simulink model "PanelSolarSeguidor_mk2_comp"  (R2022a)
settings: Solver=VariableStepAuto  StartTime=0.0  StopTime=14  RelTol=1e-3
model workspace (MAT data in the model file):
  Sig = Simulink.Signal
  Sig.DataType = 'auto'
  Sig.DocUnits = 'deg'
  Sig.Dimensions = -1
  Sig.DimensionsMode = 'auto'
  Sig.Complexity = 'auto'
  Sig.SampleTime = -1
  Sig.SamplingMode = 'auto'
values from neighbouring files (symbols this model uses):
  dia = 1    [PanelSolarSeguidor_3D.m]
  dph = 0.35    [PanelSolarSeguidor_3D.m]
  eficiencia_custom = 10    [PanelSolarSeguidor_3D.m]
  G_retroceso = -20    [PanelSolarSeguidor_3D.m]
  hra = 1    [PanelSolarSeguidor_3D.m]
  Kd = 5    [PanelSolarSeguidor.mat]    (also in PanelSolarSeguidor_3D.m)
  Kf = 1.835    [PanelSolarSeguidor.mat]    (also in PanelSolarSeguidor_3D.m)
  Kg = 20    [PanelSolarSeguidor.mat]    (also in PanelSolarSeguidor_3D.m)
  Kt = 1.835    [PanelSolarSeguidor.mat]    (also in PanelSolarSeguidor_3D.m)
  L = 0.1042    [PanelSolarSeguidor.mat]    (also in PanelSolarSeguidor_3D.m)
  latitud = -36.83078129680368    (= -36.8307812968)    [PanelSolarSeguidor_3D.m]
  longitud = -73.0368870295651    (= -73.0368870296)    [PanelSolarSeguidor_3D.m]
  m = 24.5    [PanelSolarSeguidor.mat]
  mes = 1    [PanelSolarSeguidor_3D.m]
  mn = 0    [PanelSolarSeguidor_3D.m]
  P_L = 2.18    [PanelSolarSeguidor_3D.m]
  P_W = 0.996    [PanelSolarSeguidor_3D.m]
  R = 3.05    [PanelSolarSeguidor.mat]    (also in PanelSolarSeguidor_3D.m)
  S_l = 0.2    [PanelSolarSeguidor_3D.m]
  S_w = 0.1    [PanelSolarSeguidor_3D.m]
  secs = 0    [PanelSolarSeguidor_3D.m]
  selector_eficiencia = 0    [PanelSolarSeguidor_3D.m]
  timezone = -3    [PanelSolarSeguidor_3D.m]
libraries: simulink x21, simulink_extras x9, slpidlib x2
settings Model: Creator=marte  LastModifiedBy=fmartel2019
settings ModelReferenceCC: EnableRefExpFcnMdlSchedulingChecks=off
settings RTWCC: Description=Generic Real-Time Target

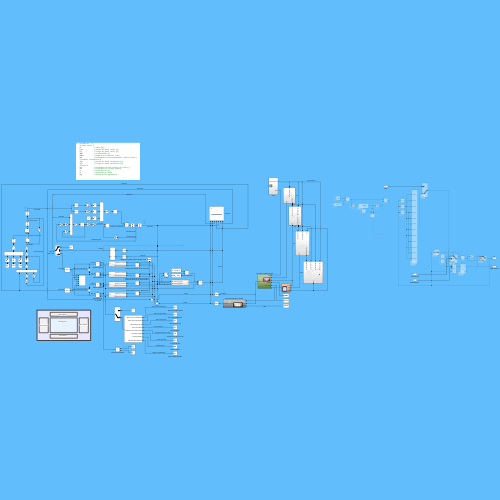
[thumbnail: Simulink's stored preview of the top-level diagram]
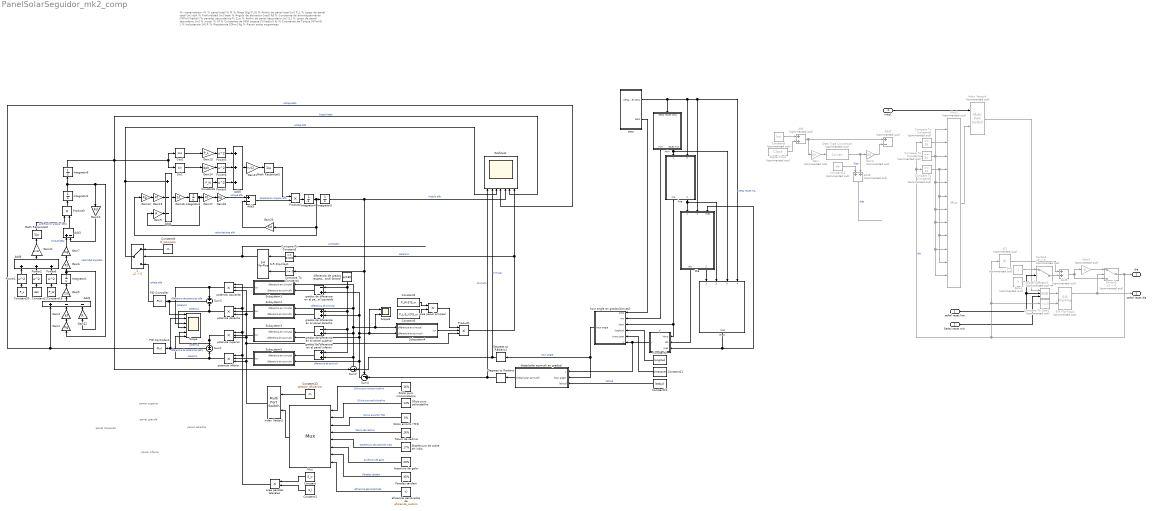
== system PanelSolarSeguidor_mk2_comp ==
  note: %---parametros---%
      | % panel total %
      | M % Masa [Kg]
      | P_W % Ancho de panel total [m]
      | P_L % Largo de panel total [m]
      | dph % Profundidad [m]
      | beta % Ángulo de elevación [rad]
      | Kd % Constante de amortiguamiento [(N*m)/(rad/s)]
      | %-paneles secundarios-%
      | S_w % Ancho de panel secundario [m]
      | S_l % Largo de panel secundario [m]
      | % motor %
      | Kf % Constante de FEM trasera [V/(rad/s)]
      | Kt % Constante de Torque [N*m/A]
      | L % Inductancia [H]
      | R % Resistencia [Ohm]
      | Kg % Razón entre engranajes
  note: panel superior
  note: panel inferior
  note: panel derecho
  note: panel izquierdo
  note: panel grande
  señal reset hra : Inport
  Señal reset min : Inport  Port=2
  mes1 : Inport  Port=3
  1 : Switch  Criteria=u2 > Threshold  SaturateOnIntegerOverflow=off  InputSameDT=off
  Add : Sum  Commented=on
  Add1 : Sum  Inputs=+-
  Add2 : Sum  Inputs=+--
  Add3 : Sum  Inputs=+-
  Add4 : Sum  Inputs=+--
  Add5 : Sum  Inputs=+++
  Add6 : Sum  Inputs=+++
  Add7 : Sum  Commented=on  Inputs=+-
  Add8 : Sum  Commented=on
  Add9 : Sum  Commented=on
  "Arseniuro de galio " : Constant  Value=20%
  Compare To Constant3 : simulink/Logic and Bit Operations/Compare To Constant  Commented=on  relop===  const=31  OutDataTypeStr=boolean
  Compare To Constant4 : simulink/Logic and Bit Operations/Compare To Constant  relop=<=  const=0  OutDataTypeStr=boolean
  Compare To Constant5 : simulink/Logic and Bit Operations/Compare To Constant  relop=<=  const=0.001  OutDataTypeStr=boolean
  Compare To Constant6 : simulink/Logic and Bit Operations/Compare To Constant  Commented=on  relop===  const=28  OutDataTypeStr=boolean
  Compare To Constant8 : simulink/Logic and Bit Operations/Compare To Constant  Commented=on  relop===  const=31  OutDataTypeStr=boolean
  Compare To Zero2 : simulink/Logic and Bit Operations/Compare To Zero  Commented=on  relop=<=  OutDataTypeStr=boolean
  Constant : Constant  Value=S_w
  Constant1 : Constant  Value=S_l
  Constant10 : Constant  Value=latitud
  Constant11 : Constant  Value=timezone
  Constant12 : Constant  Commented=on  Value=dia
  Constant13 : Constant  Value=selector_eficiencia
  Constant19 : Constant  Value=P_W
  Constant2 : Constant  Value=P_W-2*S_w
  Constant20 : Constant  Value=P_L
  Constant23 : Constant  Value=dph
  Constant3 : Constant  Value=P_L-S_l-2*S_w
  Constant4 : Constant  Value=longitud
  Constant5 : Constant  Commented=on  Value=hra
  Constant6 : Constant  Value=P_W
  Constant9 : Constant  Value=G_retroceso
  Cos1 : Trigonometry  Operator=cos
  Data Type Conversion : DataTypeConversion  Commented=on  SaturateOnIntegerOverflow=off  RndMeth=Floor
  Degrees to Radians : simulink_extras/Transformations/Degrees to Radians
  Degrees to Radians1 : simulink_extras/Transformations/Degrees to Radians
  Dia : Subsystem
  Digital Clock : DigitalClock  Commented=on
  Diseleniuro de cobre en indio : Constant  Value=17%
  Gain : Gain  Commented=on  Gain=1/24
  Gain{1,7,12,18} (4 alike) : Gain  Gain=Kg
  Gain10 : Gain  Gain=Kd
  Gain11 : Gain  Gain=m/12
  Gain13 : Gain  Gain=P_L
  Gain14 : Gain  Gain=dph
  Gain15 : Gain  Gain=Kf
  Gain16 : Gain  Gain=1/L
  Gain17 : Gain  Gain=Kt
  Gain2 : Gain  Commented=on  Gain=24
  Gain20 : Gain  Gain=Kd
  Gain21 : Gain  Gain=m/12
  Gain22 : Gain  Gain=R
  Gain3 : Gain  Commented=on  Gain=0
  Gain4 : Gain  Gain=Kf
  Gain5 : Gain  Gain=1/L
  Gain6 : Gain  Gain=Kt
  Gain9 : Gain  Gain=R
  Graficos1 : Scope  NumInputPorts=7
  IC2 : InitialCondition  Commented=on  Value=dia
  Index Vector2 : MultiPortSwitch  DataPortOrder=Zero-based contiguous  Inputs=1  zeroidx=on  SaturateOnIntegerOverflow=off  InputSameDT=off
  Index Vector4 : MultiPortSwitch  Commented=on  DataPortOrder=Zero-based contiguous  Inputs=1  zeroidx=on  SaturateOnIntegerOverflow=off  InputSameDT=off
  Integrator{1..6} (6 alike) : Integrator
  Logical Operator1 : Logic  Commented=on  Inputs=3  AllPortsSameDT=off  OutDataTypeStr=boolean
  Math Reciprocal1 : Math  Operator=reciprocal  SignedPower=on
  Math Reciprocal2 : Math  Operator=reciprocal  SignedPower=on
  Mux : Mux  Inputs=8
      settings: DisplayOption=signals
  Mux3 : Mux  Commented=on  Inputs=12
      settings: DisplayOption=signals
  One : Constant  Commented=on  OutDataTypeStr=Inherit: Inherit via back propagation
  PID Controller : slpidlib/PID Controller  Controller=P  Form=Parallel  TimeDomain=Continuous-time  UseExternalTs=off  SampleTime=-1  IntegratorMethod=Forward Euler  FilterMethod=Forward Euler  ControllerParametersSource=internal  P=10  I=0  UseKiTs=off  D=15  N=100  UseFilter=on  TunerSelectOption=Transfer Function Based (PID Tuner App)  InitialConditionSource=internal  InitialConditionForIntegrator=0  InitialConditionForFilter=0  DifferentiatorICPrevScaledInput=0  ExternalReset=none  TrackingMode=off  Kt=1  LimitOutput=off  SatLimitsSource=internal  UpperSaturationLimit=inf  LowerSaturationLimit=-inf  LinearizeAsGain=on  AntiWindupMode=none  Kb=1  POutMin=[]  POutMax=[]  IOutMin=[]  IOutMax=[]  DOutMin=[]  DOutMax=[]  NOutMin=[]  NOutMax=[]  SumOutMin=[]  SumOutMax=[]  SaturationOutMin=[]  SaturationOutMax=[]  PParamMin=[]  PParamMax=[]  IParamMin=[]  IParamMax=[]  DParamMin=[]  DParamMax=[]  NParamMin=[]  NParamMax=[]  KbParamMin=[]  KbParamMax=[]  KtParamMin=[]  KtParamMax=[]  KbOutMin=[]  KbOutMax=[]  KtOutMin=[]  KtOutMax=[]  IntegratorOutMin=[]  IntegratorOutMax=[]  FilterOutMin=[]  FilterOutMax=[]  SumI1OutMin=[]  SumI1OutMax=[]  SumI2OutMin=[]  SumI2OutMax=[]  SumI3OutMin=[]  SumI3OutMax=[]  SumI4OutMin=[]  SumI4OutMax=[]  SumDOutMin=[]  SumDOutMax=[]  DifferentiatorOutMin=[]  DifferentiatorOutMax=[]  FilterDiffOutCoefMin=[]  FilterDiffOutCoefMax=[]  ReciprocalOutMin=[]  ReciprocalOutMax=[]  SumDenOutMin=[]  SumDenOutMax=[]  SumNumOutMin=[]  SumNumOutMax=[]  DivideOutMin=[]  DivideOutMax=[]  UdiffTsProdOutMin=[]  UdiffTsProdOutMax=[]  NTsProdOutMin=[]  NTsProdOutMax=[]  UintegralTsProdOutMin=[]  UintegralTsProdOutMax=[]  UngainTsProdOutMin=[]  UngainTsProdOutMax=[]  IntegratorContinuousStateAttributes=''  IntegratorStateMustResolveToSignalObject=off  IntegratorRTWStateStorageClass=Auto  FilterContinuousStateAttributes=''  FilterStateMustResolveToSignalObject=off  FilterRTWStateStorageClass=Auto  ParallelPVariant=InternalParameters  IdealPVariant=Disabled  IVariant=Disabled  DVariant=Disabled  IntegratorVariant=Disabled  SatVariant=Disabled  AWVariant=Disabled  PCopyVariant=Disabled  TRVariant=Disabled  FdbkBlocksVariant=Forward  IdealPFdbkVariant=Disabled  SatFdbkVariant=Disabled  DerivativeFilterVariant=Disabled  NVariant=Disabled  NCopyVariant=Disabled_SignalSpec  FilterICVariant=Disabled  IntegratorICVariant=Disabled  ExternalResetVariant=Disabled  TRSumVariant=Passthrough  SumFdbkVariant=Disabled  SumVariant=Passthrough_P  TsampFilterVariant=InternalTs  TsampNgainVariant=Passthrough  TsampIntegralVariant=Disabled_SignalSpec  ExternalSaturationOutDataTypeStr=Inherit: Same as second input  aMode=0
  PID Controller1 : slpidlib/PID Controller  Controller=P  Form=Parallel  TimeDomain=Continuous-time  UseExternalTs=off  SampleTime=-1  IntegratorMethod=Forward Euler  FilterMethod=Forward Euler  ControllerParametersSource=internal  P=1  I=0  UseKiTs=off  D=0  N=100  UseFilter=on  TunerSelectOption=Transfer Function Based (PID Tuner App)  InitialConditionSource=internal  InitialConditionForIntegrator=0  InitialConditionForFilter=0  DifferentiatorICPrevScaledInput=0  ExternalReset=none  TrackingMode=off  Kt=1  LimitOutput=off  SatLimitsSource=internal  UpperSaturationLimit=inf  LowerSaturationLimit=-inf  LinearizeAsGain=on  AntiWindupMode=none  Kb=1  POutMin=[]  POutMax=[]  IOutMin=[]  IOutMax=[]  DOutMin=[]  DOutMax=[]  NOutMin=[]  NOutMax=[]  SumOutMin=[]  SumOutMax=[]  SaturationOutMin=[]  SaturationOutMax=[]  PParamMin=[]  PParamMax=[]  IParamMin=[]  IParamMax=[]  DParamMin=[]  DParamMax=[]  NParamMin=[]  NParamMax=[]  KbParamMin=[]  KbParamMax=[]  KtParamMin=[]  KtParamMax=[]  KbOutMin=[]  KbOutMax=[]  KtOutMin=[]  KtOutMax=[]  IntegratorOutMin=[]  IntegratorOutMax=[]  FilterOutMin=[]  FilterOutMax=[]  SumI1OutMin=[]  SumI1OutMax=[]  SumI2OutMin=[]  SumI2OutMax=[]  SumI3OutMin=[]  SumI3OutMax=[]  SumI4OutMin=[]  SumI4OutMax=[]  SumDOutMin=[]  SumDOutMax=[]  DifferentiatorOutMin=[]  DifferentiatorOutMax=[]  FilterDiffOutCoefMin=[]  FilterDiffOutCoefMax=[]  ReciprocalOutMin=[]  ReciprocalOutMax=[]  SumDenOutMin=[]  SumDenOutMax=[]  SumNumOutMin=[]  SumNumOutMax=[]  DivideOutMin=[]  DivideOutMax=[]  UdiffTsProdOutMin=[]  UdiffTsProdOutMax=[]  NTsProdOutMin=[]  NTsProdOutMax=[]  UintegralTsProdOutMin=[]  UintegralTsProdOutMax=[]  UngainTsProdOutMin=[]  UngainTsProdOutMax=[]  IntegratorContinuousStateAttributes=''  IntegratorStateMustResolveToSignalObject=off  IntegratorRTWStateStorageClass=Auto  FilterContinuousStateAttributes=''  FilterStateMustResolveToSignalObject=off  FilterRTWStateStorageClass=Auto  ParallelPVariant=InternalParameters  IdealPVariant=Disabled  IVariant=Disabled  DVariant=Disabled  IntegratorVariant=Disabled  SatVariant=Disabled  AWVariant=Disabled  PCopyVariant=Disabled  TRVariant=Disabled  FdbkBlocksVariant=Forward  IdealPFdbkVariant=Disabled  SatFdbkVariant=Disabled  DerivativeFilterVariant=Disabled  NVariant=Disabled  NCopyVariant=Disabled_SignalSpec  FilterICVariant=Disabled  IntegratorICVariant=Disabled  ExternalResetVariant=Disabled  TRSumVariant=Passthrough  SumFdbkVariant=Disabled  SumVariant=Passthrough_P  TsampFilterVariant=InternalTs  TsampNgainVariant=Passthrough  TsampIntegralVariant=Disabled_SignalSpec  ExternalSaturationOutDataTypeStr=Inherit: Same as second input  aMode=0
  Paneles tándem : Constant  Value=35%
  Power{1..6} (6 alike) : Math  Operator=square
  Product1 : Product  Inputs=3
  Product3 : Product
  Product4 : Product
  S-R Flip-Flop1 : simulink_extras/Flip Flops/S-R Flip-Flop  initial_condition=0
  S-R Flip-Flop4 : simulink_extras/Flip Flops/S-R Flip-Flop  Commented=on  initial_condition=0
  Scope : Scope  NumInputPorts=6
  Scope3 : Scope  NumInputPorts=2
  Silicio amorfo (TFS) : Constant  Value=5%
  Silicio puro monocristalino : Constant  Value=16%
  Silicio puro policristalino : Constant  Value=14%
  Sin1 : Trigonometry
  Subsystem1 : Subsystem
  Subsystem2 : Subsystem
  Subsystem3 : Subsystem
  Subsystem4 : Subsystem
  Subsystem5 : Subsystem
  Sum1 : Sum  Inputs=+|-
  Sum2 : Sum  Inputs=-|+
  Sum3 : Sum  Inputs=+|-
  Sum4 : Sum  Inputs=-+|
  Switch2 : Switch  Commented=on  Criteria=u2 > Threshold  SaturateOnIntegerOverflow=off  InputSameDT=off
  Switch4 : Switch  Commented=on  Criteria=u2 > Threshold  SaturateOnIntegerOverflow=off  InputSameDT=off
  "Teluro de cadmio " : Constant  Value=16%
  Zero1 : Constant  Commented=on  Value=0  OutDataTypeStr=Inherit: Inherit via back propagation
  area panel principal : Product
  area paneles laterales : Product
  diferencia de grados respecto al panel central : Constant  Value=pi/180
  eficiencia personalizada : Constant  Value=eficiencia_custom
  grados de diferencia en el panel derecho : Sum
  grados de diferencia en el panel inferior : Sum
  grados de diferencia en el panel izquierdo : Sum  Inputs=-+
  grados de diferencia en el panel superior : Sum  Inputs=-+
  hour angle en grados(cimutal) : Subsystem
  hra : Subsystem
  mes : Subsystem
  min : Subsystem
  potencia derecha : Product  Inputs=3
  potencia inferior : Product  Inputs=3
  potencia izquierda : Product  Inputs=3
  potencia superior : Product  Inputs=3
  secs : Subsystem
  theta(solar azimuth en grados) : Subsystem
  y : Subsystem
  dia : Outport
  señal reset dia : Outport  Port=2
  wires:
  hour angle en grados(cimutal)/1(hour angle) -> Degrees to Radians1/1, theta(solar azimuth en grados)/2(hour angle)  "hour angle"
  Gain12/1 -> Gain15/1
  potencia izquierda/1 -> Sum3/1, Scope/3  "potencia"
  Power5/1 -> Add5/3
  Product1/1 -> Compare To Constant5/1, Graficos1/7  "potencia"
  Power3/1 -> Add5/1
  Add5/1 -> Gain21/1
  Gain9/1 -> Add4/3
  Gain16/1 -> Integrator3/1
  Compare To Constant5/1 -> S-R Flip-Flop1/1
  potencia derecha/1 -> Sum3/2, Scope/4  "potencia"
  S-R Flip-Flop1/1 -> 1/2  "Limpiador"
  Integrator5/1 -> Graficos1/5, Sum4/1, Compare To Constant4/1  "Angulo alfa"
  Gain15/1 -> Add4/2
  Product4/1 -> Integrator4/1
  Constant9/1 -> 1/1
  Gain18/1 -> Add3/1  "torque alfa"
  Gain21/1 -> Math Reciprocal1/1
  Sin1/1 -> Gain14/1
  Math Reciprocal1/1 -> Product4/1
  Sum4/1 -> Subsystem5/2(diferencia en azimuth), grados de diferencia en el panel izquierdo/2, grados de diferencia en el panel derecho/2, Scope3/1, Subsystem4/2(diferencia en azimuth), Subsystem3/2(diferencia en azimuth)  "diferencia de azimutl"
  Gain14/1 -> Power4/1
  Power4/1 -> Add5/2
  Cos1/1 -> Gain13/1
  Add4/1 -> Gain16/1
  Add3/1 -> Product4/2  "aceleracion angular alfa"
  Gain17/1 -> Gain18/1
  Subsystem1/1(lux) -> potencia izquierda/2
  Gain20/1 -> Add3/2
  Integrator3/1 -> Gain17/1, Gain9/1
  Compare To Constant4/1 -> S-R Flip-Flop1/2
  Integrator4/1 -> Gain12/1, Gain20/1, Integrator5/1  "velocidad ang alfa"
  Sum3/1 -> PID Controller/1, Scope/1  "diferencia de potencias alfa"
  Constant6/1 -> Power5/1
  Gain13/1 -> Power3/1
  eficiencia personalizada/1 -> Mux/8  "eficiencia personalizada"
  Silicio puro monocristalino/1 -> Mux/1  "Silicio puro monocristalino"
  Silicio puro policristalino/1 -> Mux/2  "Silicio puro policristalino"
  Silicio amorfo (TFS)/1 -> Mux/3  "Silicio amorfo (TFS)"
  "Teluro de cadmio "/1 -> Mux/4  "Teluro de cadmio"
  Diseleniuro de cobre en indio/1 -> Mux/5  "Diseleniuro de cobre en indio"
  "Arseniuro de galio "/1 -> Mux/6  "Arseniuro de galio"
  Paneles tándem/1 -> Mux/7  "Paneles tándem"
  Mux/1 -> Index Vector2/2
  Constant13/1 -> Index Vector2/1
  Constant/1 -> area paneles laterales/1
  Constant1/1 -> area paneles laterales/2
  Subsystem4/1(lux) -> Product1/2
  Subsystem2/1(lux) -> potencia derecha/2
  grados de diferencia en el panel izquierdo/1 -> Subsystem1/2(diferencia en azimuth)
  grados de diferencia en el panel derecho/1 -> Subsystem2/2(diferencia en azimuth)
  Constant3/1 -> area panel principal/2
  Constant2/1 -> area panel principal/1
  area panel principal/1 -> Product1/1
  y/1(y) -> hour angle en grados(cimutal)/6(y), theta(solar azimuth en grados)/1(y)
  Constant10/1 -> theta(solar azimuth en grados)/3(latitud)  "latitud"
  Constant4/1 -> hour angle en grados(cimutal)/4(longitud)
  Constant11/1 -> hour angle en grados(cimutal)/5(time zone)
  theta(solar azimuth en grados)/1(theta(solar azimuth)) -> Degrees to Radians/1
  grados de diferencia en el panel superior/1 -> Subsystem3/1(diferencia en cimutal)
  Gain7/1 -> Add1/1  "torque beta"
  grados de diferencia en el panel inferior/1 -> Subsystem5/1(diferencia en cimutal)
  1/1 -> Add4/1, Graficos1/3  "voltaje alfa"
  diferencia de grados respecto al panel central/1 -> grados de diferencia en el panel izquierdo/1, grados de diferencia en el panel derecho/1, grados de diferencia en el panel superior/1, grados de diferencia en el panel inferior/1
  Gain4/1 -> Add2/2
  Gain11/1 -> Math Reciprocal2/1
  area paneles laterales/1 -> potencia izquierda/1, potencia derecha/1, potencia superior/1, potencia inferior/1
  Gain6/1 -> Gain7/1
  Subsystem5/1(lux) -> potencia inferior/2
  Index Vector2/1 -> Product1/3, potencia superior/3, potencia izquierda/3, potencia derecha/3, potencia inferior/3
  Add1/1 -> Product3/2  "aceleracion angular beta"
  Constant20/1 -> Power1/1
  Constant19/1 -> Power6/1
  Integrator1/1 -> Gain6/1, Gain22/1
  Sum1/1 -> Scope/2, PID Controller1/1  "diferencia de potencias beta"
  Sum2/1 -> Subsystem1/1(diferencia en cimutal), Subsystem2/1(diferencia en cimutal), Scope3/2, Subsystem4/1(diferencia en cimutal), grados de diferencia en el panel superior/2, grados de diferencia en el panel inferior/2  "diferencia de cimutal"
  Integrator2/1 -> Gain10/1, Gain1/1, Integrator6/1  "velocidad ang beta"
  Gain10/1 -> Add1/2
  Gain5/1 -> Integrator1/1
  Gain22/1 -> Add2/3
  Add2/1 -> Gain5/1
  Constant23/1 -> Power2/1
  Integrator6/1 -> Graficos1/6, Cos1/1, Sin1/1, Sum2/1  "Angulo beta"
  Power2/1 -> Add6/2
  Subsystem3/1(lux) -> potencia superior/2
  Power6/1 -> Add6/3
  Math Reciprocal2/1 -> Product3/1
  Power1/1 -> Add6/1
  Product3/1 -> Integrator2/1
  Add6/1 -> Gain11/1
  potencia inferior/1 -> Scope/6, Sum1/2  "potencia"
  Gain1/1 -> Gain4/1
  potencia superior/1 -> Scope/5, Sum1/1  "potencia"
  secs/1(señal reset secs) -> mes/4(Señal reset secs), Dia/2(Señal reset min), hra/2(Señal reset secs), min/1(Señal reset secs)  "señal reset hra"
  Dia/2(señal reset dia) -> mes/1("Señal reset dia ")
  hra/2(Señal reset hra) -> Dia/1(señal reset hra), mes/2(señal reset hra)
  min/2(reset min) -> mes/3(Señal reset min), hra/1(Señal reset mins)
  Degrees to Radians/1 -> Sum4/2, Graficos1/1  "azimuth"
  Degrees to Radians1/1 -> Sum2/2, Graficos1/2  "cimutal"
  Constant5/1 -> Add/1
  Digital Clock/1 -> Add/2
  Add/1 -> Gain/1, Add7/1
  Gain/1 -> Data Type Conversion/1
  Data Type Conversion/1 -> Add8/2, Gain2/1  "Dias"
  Gain2/1 -> Add7/2
  Constant12/1 -> Add8/1
  Add8/1 -> ?  "dias"
  Compare To Constant3/1 -> Mux3/12, Mux3/10, Mux3/8, Mux3/7, Mux3/5, Mux3/1, Mux3/3
  Señal reset min/1 -> Logical Operator1/3
  Zero1/1 -> Switch4/3
  Gain3/1 -> Switch2/1
  One/1 -> Switch4/1
  Compare To Constant8/1 -> Mux3/11, Mux3/9, Mux3/6, Mux3/4
  Switch2/1 -> dia/1, Compare To Constant3/1, Compare To Constant6/1, Compare To Constant8/1, IC2/1, Compare To Zero2/1  "dia"
  Compare To Zero2/1 -> S-R Flip-Flop4/2
  Add9/1 -> Switch2/3, Gain3/1
  Switch4/1 -> Add9/2
  Mux3/1 -> Index Vector4/2
  Compare To Constant6/1 -> Mux3/2
  mes1/1 -> Index Vector4/1
  Index Vector4/1 -> Logical Operator1/1
  señal reset hra/1 -> Switch4/2, Logical Operator1/2
  S-R Flip-Flop4/1 -> Switch2/2, señal reset dia/1
  Logical Operator1/1 -> S-R Flip-Flop4/1
  IC2/1 -> Add9/1
  PID Controller1/1 -> Add2/1, Graficos1/4  "voltaje beta"
  secs/2(Secs) -> hour angle en grados(cimutal)/1(secs)
  min/1(min) -> hour angle en grados(cimutal)/2(mn)
  hra/1(hra) -> hour angle en grados(cimutal)/3(hora), y/1(Hora)
  Dia/1(dia) -> y/2(dia)
  mes/1(mes) -> Dia/3(mes), y/3(mes)
  PID Controller/1 -> 1/3  "voltaje alfa"

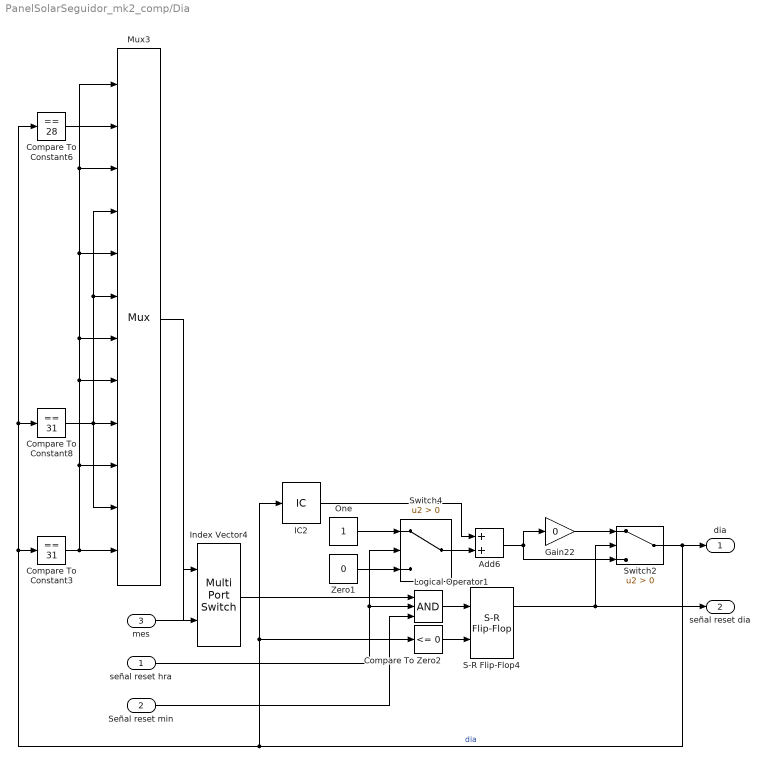
== system PanelSolarSeguidor_mk2_comp/Dia ==
  señal reset hra : Inport
  Señal reset min : Inport  Port=2
  mes : Inport  Port=3
  Add6 : Sum
  Compare To Constant3 : simulink/Logic and Bit Operations/Compare To Constant  relop===  const=31  OutDataTypeStr=boolean
  Compare To Constant6 : simulink/Logic and Bit Operations/Compare To Constant  relop===  const=28  OutDataTypeStr=boolean
  Compare To Constant8 : simulink/Logic and Bit Operations/Compare To Constant  relop===  const=31  OutDataTypeStr=boolean
  Compare To Zero2 : simulink/Logic and Bit Operations/Compare To Zero  relop=<=  OutDataTypeStr=boolean
  Gain22 : Gain  Gain=0
  IC2 : InitialCondition  Value=dia
  Index Vector4 : MultiPortSwitch  DataPortOrder=Zero-based contiguous  Inputs=1  zeroidx=on  SaturateOnIntegerOverflow=off  InputSameDT=off
  Logical Operator1 : Logic  Inputs=3  AllPortsSameDT=off  OutDataTypeStr=boolean
  Mux3 : Mux  Inputs=12
      settings: DisplayOption=signals
  One : Constant  OutDataTypeStr=Inherit: Inherit via back propagation
  S-R Flip-Flop4 : simulink_extras/Flip Flops/S-R Flip-Flop  initial_condition=0
  Switch2 : Switch  Criteria=u2 > Threshold  SaturateOnIntegerOverflow=off  InputSameDT=off
  Switch4 : Switch  Criteria=u2 > Threshold  SaturateOnIntegerOverflow=off  InputSameDT=off
  Zero1 : Constant  Value=0  OutDataTypeStr=Inherit: Inherit via back propagation
  dia : Outport
  señal reset dia : Outport  Port=2
  wires:
  Zero1/1 -> Switch4/3
  Compare To Zero2/1 -> S-R Flip-Flop4/2
  Add6/1 -> Switch2/3, Gain22/1
  S-R Flip-Flop4/1 -> Switch2/2, señal reset dia/1
  Compare To Constant8/1 -> Mux3/11, Mux3/4, Mux3/6, Mux3/9
  Compare To Constant3/1 -> Mux3/8, Mux3/1, Mux3/3, Mux3/5, Mux3/7, Mux3/10, Mux3/12
  Logical Operator1/1 -> S-R Flip-Flop4/1
  Switch2/1 -> dia/1, Compare To Constant8/1, Compare To Constant6/1, Compare To Constant3/1, IC2/1, Compare To Zero2/1  "dia"
  Mux3/1 -> Index Vector4/2
  One/1 -> Switch4/1
  Gain22/1 -> Switch2/1
  IC2/1 -> Add6/1
  Index Vector4/1 -> Logical Operator1/1
  Compare To Constant6/1 -> Mux3/2
  Switch4/1 -> Add6/2
  mes/1 -> Index Vector4/1
  señal reset hra/1 -> Switch4/2, Logical Operator1/2
  Señal reset min/1 -> Logical Operator1/3

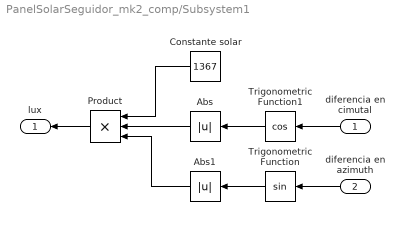
== system PanelSolarSeguidor_mk2_comp/Subsystem1 ==
  diferencia en cimutal : Inport
  diferencia en azimuth : Inport  Port=2
  Abs : Abs  SaturateOnIntegerOverflow=off
  Abs1 : Abs  SaturateOnIntegerOverflow=off
  Constante solar : Constant  Value=1367
  Product : Product  Inputs=3
  Trigonometric Function : Trigonometry
  Trigonometric Function1 : Trigonometry  Operator=cos
  lux : Outport
  wires:
  Trigonometric Function1/1 -> Abs/1
  Constante solar/1 -> Product/1
  Trigonometric Function/1 -> Abs1/1
  Product/1 -> lux/1
  diferencia en cimutal/1 -> Trigonometric Function1/1
  diferencia en azimuth/1 -> Trigonometric Function/1
  Abs1/1 -> Product/3
  Abs/1 -> Product/2

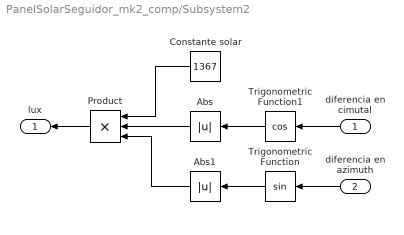
== system PanelSolarSeguidor_mk2_comp/Subsystem2 ==
  diferencia en cimutal : Inport
  diferencia en azimuth : Inport  Port=2
  Abs : Abs  SaturateOnIntegerOverflow=off
  Abs1 : Abs  SaturateOnIntegerOverflow=off
  Constante solar : Constant  Value=1367
  Product : Product  Inputs=3
  Trigonometric Function : Trigonometry
  Trigonometric Function1 : Trigonometry  Operator=cos
  lux : Outport
  wires:
  Trigonometric Function1/1 -> Abs/1
  Constante solar/1 -> Product/1
  Trigonometric Function/1 -> Abs1/1
  Product/1 -> lux/1
  diferencia en cimutal/1 -> Trigonometric Function1/1
  diferencia en azimuth/1 -> Trigonometric Function/1
  Abs1/1 -> Product/3
  Abs/1 -> Product/2

== system PanelSolarSeguidor_mk2_comp/Subsystem3 ==
  diferencia en cimutal : Inport
  diferencia en azimuth : Inport  Port=2
  Abs : Abs  SaturateOnIntegerOverflow=off
  Abs1 : Abs  SaturateOnIntegerOverflow=off
  Constante solar : Constant  Value=1367
  Product : Product  Inputs=3
  Trigonometric Function : Trigonometry
  Trigonometric Function1 : Trigonometry  Operator=cos
  lux : Outport
  wires:
  Trigonometric Function1/1 -> Abs/1
  Constante solar/1 -> Product/1
  Trigonometric Function/1 -> Abs1/1
  Product/1 -> lux/1
  diferencia en cimutal/1 -> Trigonometric Function1/1
  diferencia en azimuth/1 -> Trigonometric Function/1
  Abs1/1 -> Product/3
  Abs/1 -> Product/2

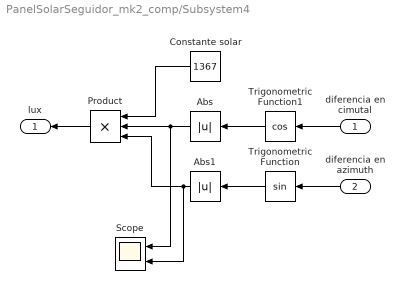
== system PanelSolarSeguidor_mk2_comp/Subsystem4 ==
  diferencia en cimutal : Inport
  diferencia en azimuth : Inport  Port=2
  Abs : Abs  SaturateOnIntegerOverflow=off
  Abs1 : Abs  SaturateOnIntegerOverflow=off
  Constante solar : Constant  Value=1367
  Product : Product  Inputs=3
  Scope : Scope  NumInputPorts=2
  Trigonometric Function : Trigonometry
  Trigonometric Function1 : Trigonometry  Operator=cos
  lux : Outport
  wires:
  Trigonometric Function1/1 -> Abs/1
  Constante solar/1 -> Product/1
  Trigonometric Function/1 -> Abs1/1
  Product/1 -> lux/1
  diferencia en cimutal/1 -> Trigonometric Function1/1
  diferencia en azimuth/1 -> Trigonometric Function/1
  Abs1/1 -> Scope/2, Product/3
  Abs/1 -> Scope/1, Product/2

== system PanelSolarSeguidor_mk2_comp/Subsystem5 ==
  diferencia en cimutal : Inport
  diferencia en azimuth : Inport  Port=2
  Abs : Abs  SaturateOnIntegerOverflow=off
  Abs1 : Abs  SaturateOnIntegerOverflow=off
  Constante solar : Constant  Value=1367
  Product : Product  Inputs=3
  Trigonometric Function : Trigonometry
  Trigonometric Function1 : Trigonometry  Operator=cos
  lux : Outport
  wires:
  Trigonometric Function1/1 -> Abs/1
  Constante solar/1 -> Product/1
  Trigonometric Function/1 -> Abs1/1
  Product/1 -> lux/1
  diferencia en cimutal/1 -> Trigonometric Function1/1
  diferencia en azimuth/1 -> Trigonometric Function/1
  Abs1/1 -> Product/3
  Abs/1 -> Product/2

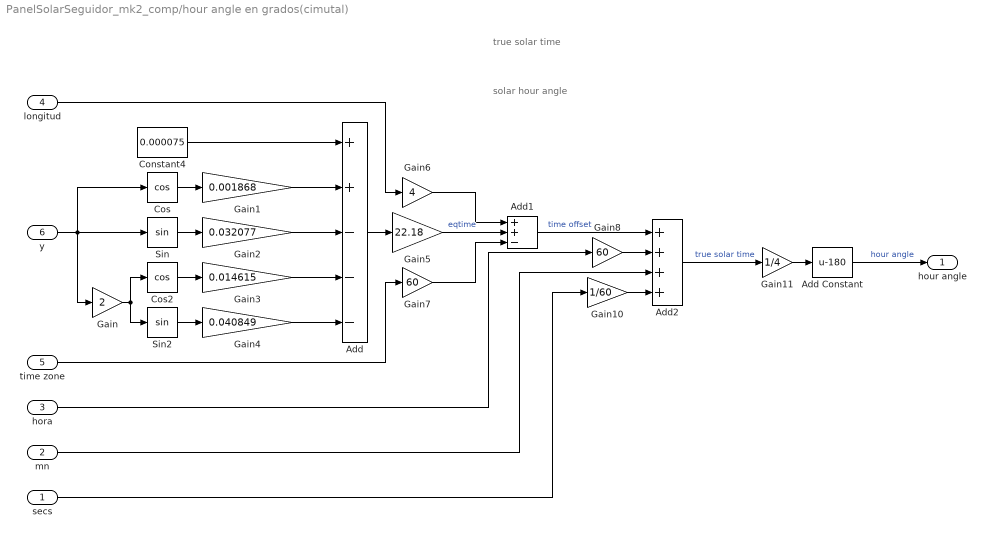
== system PanelSolarSeguidor_mk2_comp/hour angle en grados(cimutal) ==
  note: solar hour angle
  note: true solar time
  secs : Inport
  mn : Inport  Port=2
  hora : Inport  Port=3
  longitud : Inport  Port=4
  time zone : Inport  Port=5
  y : Inport  Port=6
  Add : Sum  Inputs=++---
  Add Constant : Bias  Bias=-180  SaturateOnIntegerOverflow=off
  Add1 : Sum  Inputs=++-
  Add2 : Sum  Inputs=++++
  Constant4 : Constant  Value=0.000075
  Cos : Trigonometry  Operator=cos
  Cos2 : Trigonometry  Operator=cos
  Gain : Gain  Gain=2
  Gain1 : Gain  Gain=0.001868
  Gain10 : Gain  Gain=1/60
  Gain11 : Gain  Gain=1/4
  Gain2 : Gain  Gain=0.032077
  Gain3 : Gain  Gain=0.014615
  Gain4 : Gain  Gain=0.040849
  Gain5 : Gain  Gain=22.18
  Gain6 : Gain  Gain=4
  Gain7 : Gain  Gain=60
  Gain8 : Gain  Gain=60
  Sin : Trigonometry
  Sin2 : Trigonometry
  hour angle : Outport
  wires:
  mn/1 -> Add2/3
  Gain4/1 -> Add/5
  Add1/1 -> Add2/1  "time offset"
  Cos/1 -> Gain1/1
  Cos2/1 -> Gain3/1
  Constant4/1 -> Add/1
  Gain2/1 -> Add/3
  Gain3/1 -> Add/4
  Gain8/1 -> Add2/2
  Sin/1 -> Gain2/1
  secs/1 -> Gain10/1
  Gain7/1 -> Add1/3
  Gain/1 -> Cos2/1, Sin2/1
  Gain10/1 -> Add2/4
  y/1 -> Sin/1, Gain/1, Cos/1
  longitud/1 -> Gain6/1
  Add2/1 -> Gain11/1  "true solar time"
  Gain11/1 -> Add Constant/1
  hora/1 -> Gain8/1
  Gain1/1 -> Add/2
  time zone/1 -> Gain7/1
  Add Constant/1 -> hour angle/1  "hour angle"
  Add/1 -> Gain5/1
  Gain5/1 -> Add1/2  "eqtime"
  Sin2/1 -> Gain4/1
  Gain6/1 -> Add1/1

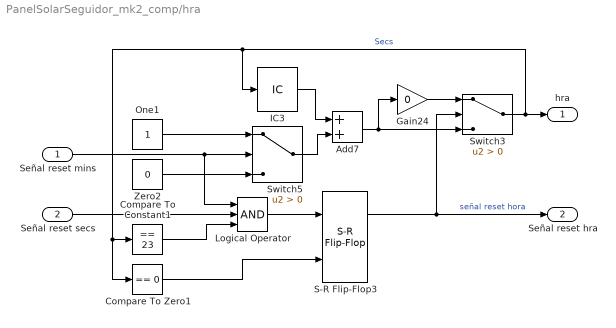
== system PanelSolarSeguidor_mk2_comp/hra ==
  Señal reset mins : Inport
  Señal reset secs : Inport  Port=2
  Add7 : Sum
  Compare To Constant1 : simulink/Logic and Bit Operations/Compare To Constant  relop===  const=23  OutDataTypeStr=boolean
  Compare To Zero1 : simulink/Logic and Bit Operations/Compare To Zero  relop===  OutDataTypeStr=boolean
  Gain24 : Gain  Gain=0
  IC3 : InitialCondition  Value=hra
  Logical Operator : Logic  Inputs=3  AllPortsSameDT=off  OutDataTypeStr=boolean
  One1 : Constant  OutDataTypeStr=Inherit: Inherit via back propagation
  S-R Flip-Flop3 : simulink_extras/Flip Flops/S-R Flip-Flop  initial_condition=0
  Switch3 : Switch  Criteria=u2 > Threshold  SaturateOnIntegerOverflow=off  InputSameDT=off
  Switch5 : Switch  Criteria=u2 > Threshold  SaturateOnIntegerOverflow=off  InputSameDT=off
  Zero2 : Constant  Value=0  OutDataTypeStr=Inherit: Inherit via back propagation
  hra : Outport
  Señal reset hra : Outport  Port=2
  wires:
  Compare To Zero1/1 -> S-R Flip-Flop3/2
  IC3/1 -> Add7/1
  Gain24/1 -> Switch3/1
  Compare To Constant1/1 -> Logical Operator/3
  Logical Operator/1 -> S-R Flip-Flop3/1
  S-R Flip-Flop3/1 -> Switch3/2, Señal reset hra/1  "señal reset hora"
  Add7/1 -> Switch3/3, Gain24/1
  One1/1 -> Switch5/1
  Zero2/1 -> Switch5/3
  Señal reset secs/1 -> Logical Operator/2
  Switch3/1 -> Compare To Constant1/1, Compare To Zero1/1, IC3/1, hra/1  "Secs"
  Señal reset mins/1 -> Logical Operator/1, Switch5/2
  Switch5/1 -> Add7/2

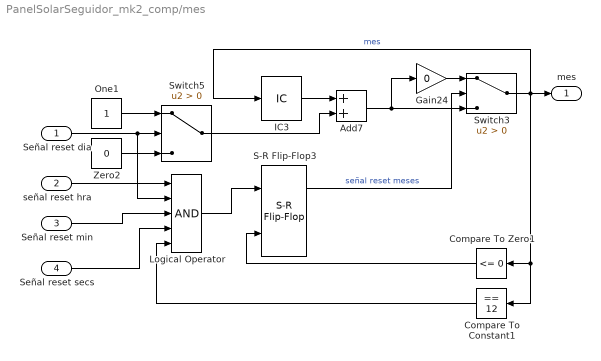
== system PanelSolarSeguidor_mk2_comp/mes ==
  "Señal reset dia " : Inport
  señal reset hra : Inport  Port=2
  Señal reset min : Inport  Port=3
  Señal reset secs : Inport  Port=4
  Add7 : Sum
  Compare To Constant1 : simulink/Logic and Bit Operations/Compare To Constant  relop===  const=12  OutDataTypeStr=boolean
  Compare To Zero1 : simulink/Logic and Bit Operations/Compare To Zero  relop=<=  OutDataTypeStr=boolean
  Gain24 : Gain  Gain=0
  IC3 : InitialCondition  Value=mes
  Logical Operator : Logic  Inputs=5  AllPortsSameDT=off  OutDataTypeStr=boolean
  One1 : Constant  OutDataTypeStr=Inherit: Inherit via back propagation
  S-R Flip-Flop3 : simulink_extras/Flip Flops/S-R Flip-Flop  initial_condition=0
  Switch3 : Switch  Criteria=u2 > Threshold  SaturateOnIntegerOverflow=off  InputSameDT=off
  Switch5 : Switch  Criteria=u2 > Threshold  SaturateOnIntegerOverflow=off  InputSameDT=off
  Zero2 : Constant  Value=0  OutDataTypeStr=Inherit: Inherit via back propagation
  mes : Outport
  wires:
  Switch3/1 -> Compare To Constant1/1, Compare To Zero1/1, IC3/1, mes/1  "mes"
  Compare To Zero1/1 -> S-R Flip-Flop3/2
  IC3/1 -> Add7/1
  "Señal reset dia "/1 -> Logical Operator/2, Switch5/2
  Gain24/1 -> Switch3/1
  Compare To Constant1/1 -> Logical Operator/5
  Logical Operator/1 -> S-R Flip-Flop3/1
  S-R Flip-Flop3/1 -> Switch3/2  "señal reset meses"
  Add7/1 -> Switch3/3, Gain24/1
  Switch5/1 -> Add7/2
  One1/1 -> Switch5/1
  Zero2/1 -> Switch5/3
  señal reset hra/1 -> Logical Operator/1
  Señal reset min/1 -> Logical Operator/3
  Señal reset secs/1 -> Logical Operator/4

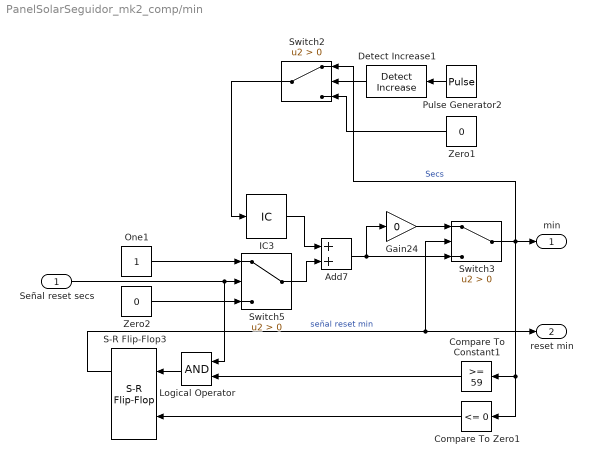
== system PanelSolarSeguidor_mk2_comp/min ==
  Señal reset secs : Inport
  Add7 : Sum
  Compare To Constant1 : simulink/Logic and Bit Operations/Compare To Constant  relop=>=  const=59  OutDataTypeStr=boolean
  Compare To Zero1 : simulink/Logic and Bit Operations/Compare To Zero  relop=<=  OutDataTypeStr=boolean
  Detect Increase1 : simulink/Logic and Bit Operations/Detect Increase  vinit=0.0  OutDataTypeStr=boolean
  Gain24 : Gain  Gain=0
  IC3 : InitialCondition  Value=mn
  Logical Operator : Logic  AllPortsSameDT=off  OutDataTypeStr=boolean
  One1 : Constant  OutDataTypeStr=Inherit: Inherit via back propagation
  Pulse Generator2 : DiscretePulseGenerator  PulseType=Time based  Period=1/60  PulseWidth=5
  S-R Flip-Flop3 : simulink_extras/Flip Flops/S-R Flip-Flop  initial_condition=0
  Switch2 : Switch  Criteria=u2 > Threshold  SaturateOnIntegerOverflow=off  InputSameDT=off
  Switch3 : Switch  Criteria=u2 > Threshold  SaturateOnIntegerOverflow=off  InputSameDT=off
  Switch5 : Switch  Criteria=u2 > Threshold  SaturateOnIntegerOverflow=off  InputSameDT=off
  Zero1 : Constant  Value=0  OutDataTypeStr=Inherit: Inherit via back propagation
  Zero2 : Constant  Value=0  OutDataTypeStr=Inherit: Inherit via back propagation
  min : Outport
  reset min : Outport  Port=2
  wires:
  Compare To Zero1/1 -> S-R Flip-Flop3/2
  IC3/1 -> Add7/1
  Señal reset secs/1 -> Switch5/2, Logical Operator/1
  Gain24/1 -> Switch3/1
  Compare To Constant1/1 -> Logical Operator/2
  Logical Operator/1 -> S-R Flip-Flop3/1
  S-R Flip-Flop3/1 -> reset min/1, Switch3/2  "señal reset min"
  Add7/1 -> Switch3/3, Gain24/1
  Switch5/1 -> Add7/2
  One1/1 -> Switch5/1
  Zero2/1 -> Switch5/3
  Detect Increase1/1 -> Switch2/2
  Pulse Generator2/1 -> Detect Increase1/1
  Zero1/1 -> Switch2/3
  Switch3/1 -> Compare To Zero1/1, Compare To Constant1/1, Switch2/1, min/1  "Secs"
  Switch2/1 -> IC3/1

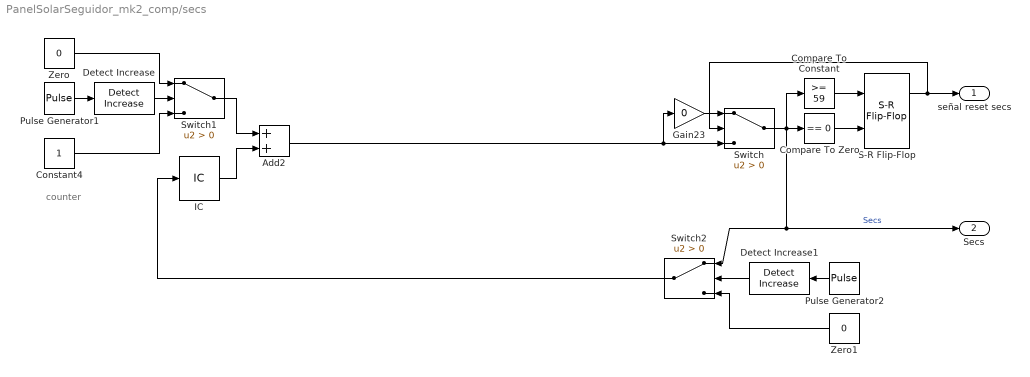
== system PanelSolarSeguidor_mk2_comp/secs ==
  note: counter
  Add2 : Sum
  Compare To Constant : simulink/Logic and Bit Operations/Compare To Constant  relop=>=  const=59  OutDataTypeStr=boolean
  Compare To Zero : simulink/Logic and Bit Operations/Compare To Zero  relop===  OutDataTypeStr=boolean
  Constant4 : Constant
  Detect Increase : simulink/Logic and Bit Operations/Detect Increase  vinit=0.0  OutDataTypeStr=boolean
  Detect Increase1 : simulink/Logic and Bit Operations/Detect Increase  vinit=0.0  OutDataTypeStr=boolean
  Gain23 : Gain  Gain=0
  IC : InitialCondition  Value=secs
  Pulse Generator1 : DiscretePulseGenerator  PulseType=Time based  Period=1/3600  PulseWidth=5
  Pulse Generator2 : DiscretePulseGenerator  PulseType=Time based  Period=1/3600  PulseWidth=5
  S-R Flip-Flop : simulink_extras/Flip Flops/S-R Flip-Flop  initial_condition=0
  Switch : Switch  Criteria=u2 > Threshold  SaturateOnIntegerOverflow=off  InputSameDT=off
  Switch1 : Switch  Criteria=u2 > Threshold  SaturateOnIntegerOverflow=off  InputSameDT=off
  Switch2 : Switch  Criteria=u2 > Threshold  SaturateOnIntegerOverflow=off  InputSameDT=off
  Zero : Constant  Value=0  OutDataTypeStr=Inherit: Inherit via back propagation
  Zero1 : Constant  Value=0  OutDataTypeStr=Inherit: Inherit via back propagation
  señal reset secs : Outport
  Secs : Outport  Port=2
  wires:
  Compare To Zero/1 -> S-R Flip-Flop/2
  Gain23/1 -> Switch/1
  Compare To Constant/1 -> S-R Flip-Flop/1
  Add2/1 -> Switch/3, Gain23/1
  S-R Flip-Flop/1 -> Switch/2, señal reset secs/1
  Switch/1 -> Compare To Constant/1, Compare To Zero/1, Switch2/1, Secs/1  "Secs"
  Pulse Generator1/1 -> Detect Increase/1
  IC/1 -> Add2/2
  Constant4/1 -> Switch1/3
  Detect Increase/1 -> Switch1/2
  Switch1/1 -> Add2/1
  Zero/1 -> Switch1/1
  Detect Increase1/1 -> Switch2/2
  Zero1/1 -> Switch2/3
  Pulse Generator2/1 -> Detect Increase1/1
  Switch2/1 -> IC/1

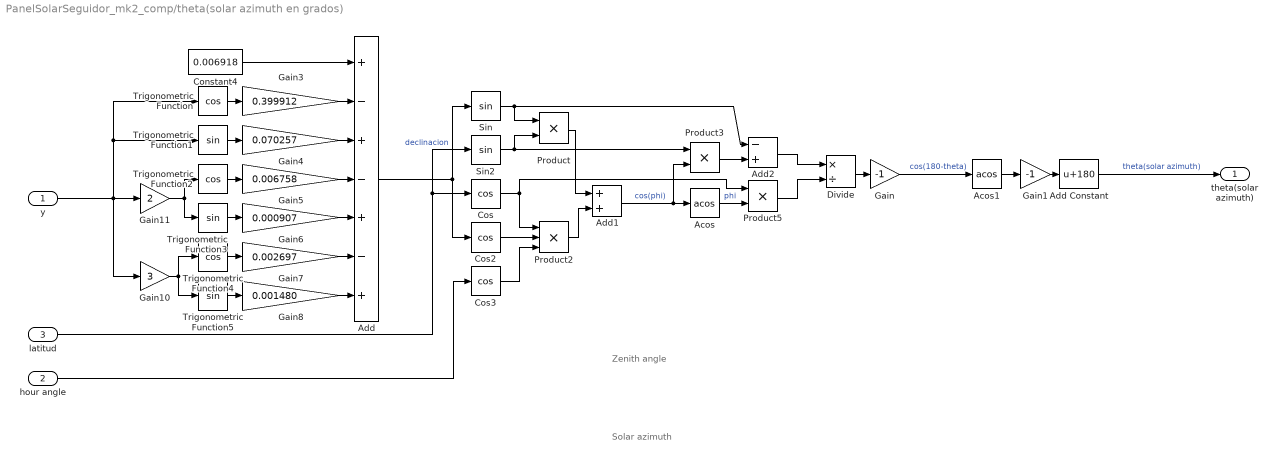
== system PanelSolarSeguidor_mk2_comp/theta(solar azimuth en grados) ==
  note: Solar azimuth
  note: Zenith angle
  y : Inport
  hour angle : Inport  Port=2
  latitud : Inport  Port=3
  Acos : Trigonometry  Operator=acos
  Acos1 : Trigonometry  Operator=acos
  Add : Sum  Inputs=+-+-+-+
  Add Constant : Bias  Bias=180  SaturateOnIntegerOverflow=off
  Add1 : Sum
  Add2 : Sum  Inputs=-+
  Constant4 : Constant  Value=0.006918
  Cos : Trigonometry  Operator=cos
  Cos2 : Trigonometry  Operator=cos
  Cos3 : Trigonometry  Operator=cos
  Divide : Product  Inputs=*/
  Gain : Gain  Gain=-1
  Gain1 : Gain  Gain=-1
  Gain10 : Gain  Gain=3
  Gain11 : Gain  Gain=2
  Gain3 : Gain  Gain=0.399912
  Gain4 : Gain  Gain=0.070257
  Gain5 : Gain  Gain=0.006758
  Gain6 : Gain  Gain=0.000907
  Gain7 : Gain  Gain=0.002697
  Gain8 : Gain  Gain=0.001480
  Product : Product
  Product2 : Product  Inputs=3
  Product3 : Product
  Product5 : Product
  Sin : Trigonometry
  Sin2 : Trigonometry
  Trigonometric Function : Trigonometry  Operator=cos
  Trigonometric Function1 : Trigonometry
  Trigonometric Function2 : Trigonometry  Operator=cos
  Trigonometric Function3 : Trigonometry
  Trigonometric Function4 : Trigonometry  Operator=cos
  Trigonometric Function5 : Trigonometry
  theta(solar azimuth) : Outport
  wires:
  Gain6/1 -> Add/5
  Gain7/1 -> Add/6
  hour angle/1 -> Cos3/1
  Acos1/1 -> Gain1/1
  Add1/1 -> Product3/2, Acos/1  "cos(phi)"
  Sin/1 -> Product/1, Add2/1
  Constant4/1 -> Add/1
  latitud/1 -> Cos/1, Sin2/1
  Gain5/1 -> Add/4
  Sin2/1 -> Product/2, Product3/1
  Add Constant/1 -> theta(solar azimuth)/1  "theta(solar azimuth)"
  y/1 -> Gain10/1, Gain11/1, Trigonometric Function/1, Trigonometric Function1/1
  Product3/1 -> Add2/2
  Product2/1 -> Add1/2
  Acos/1 -> Product5/2  "phi"
  Gain10/1 -> Trigonometric Function4/1, Trigonometric Function5/1
  Add/1 -> Sin/1, Cos2/1  "declinacion"
  Gain8/1 -> Add/7
  Trigonometric Function2/1 -> Gain5/1
  Gain11/1 -> Trigonometric Function3/1, Trigonometric Function2/1
  Trigonometric Function/1 -> Gain3/1
  Cos/1 -> Product5/1, Product2/1
  Trigonometric Function1/1 -> Gain4/1
  Cos3/1 -> Product2/3
  Add2/1 -> Divide/1
  Gain1/1 -> Add Constant/1
  Divide/1 -> Gain/1
  Gain4/1 -> Add/3
  Trigonometric Function4/1 -> Gain7/1
  Trigonometric Function3/1 -> Gain6/1
  Gain/1 -> Acos1/1  "cos(180-theta)"
  Product5/1 -> Divide/2
  Trigonometric Function5/1 -> Gain8/1
  Gain3/1 -> Add/2
  Cos2/1 -> Product2/2
  Product/1 -> Add1/1

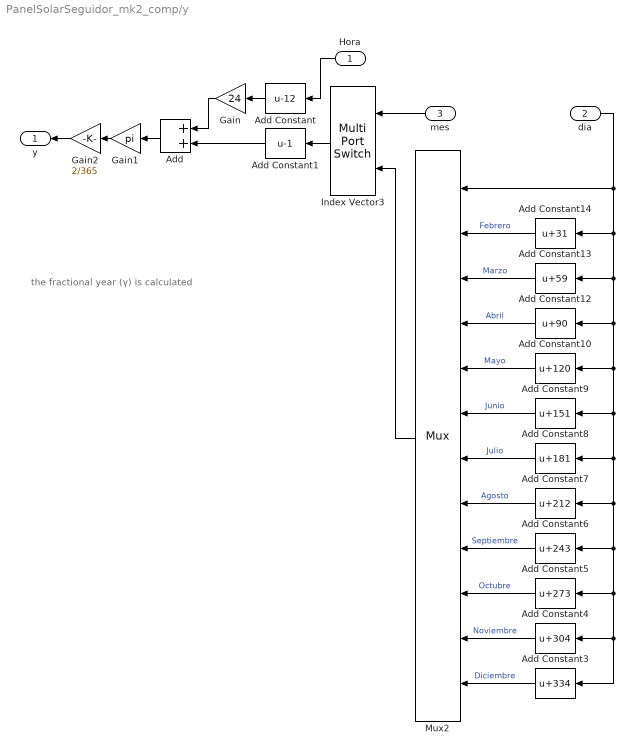
== system PanelSolarSeguidor_mk2_comp/y ==
  note: the fractional year (γ) is calculated
  Hora : Inport
  dia : Inport  Port=2
  mes : Inport  Port=3
  Add : Sum
  Add Constant : Bias  Bias=-12  SaturateOnIntegerOverflow=off
  Add Constant1 : Bias  Bias=-1  SaturateOnIntegerOverflow=off
  Add Constant10 : Bias  Bias=120  SaturateOnIntegerOverflow=off
  Add Constant12 : Bias  Bias=90  SaturateOnIntegerOverflow=off
  Add Constant13 : Bias  Bias=59  SaturateOnIntegerOverflow=off
  Add Constant14 : Bias  Bias=31  SaturateOnIntegerOverflow=off
  Add Constant3 : Bias  Bias=334  SaturateOnIntegerOverflow=off
  Add Constant4 : Bias  Bias=304  SaturateOnIntegerOverflow=off
  Add Constant5 : Bias  Bias=273  SaturateOnIntegerOverflow=off
  Add Constant6 : Bias  Bias=243  SaturateOnIntegerOverflow=off
  Add Constant7 : Bias  Bias=212  SaturateOnIntegerOverflow=off
  Add Constant8 : Bias  Bias=181  SaturateOnIntegerOverflow=off
  Add Constant9 : Bias  Bias=151  SaturateOnIntegerOverflow=off
  Gain : Gain  Gain=24
  Gain1 : Gain  Gain=pi
  Gain2 : Gain  Gain=2/365
  Index Vector3 : MultiPortSwitch  DataPortOrder=Zero-based contiguous  Inputs=1  zeroidx=on  SaturateOnIntegerOverflow=off  InputSameDT=off
  Mux2 : Mux  Inputs=12
      settings: DisplayOption=signals
  y : Outport
  wires:
  dia/1 -> Mux2/1, Add Constant12/1, Add Constant10/1, Add Constant9/1, Add Constant8/1, Add Constant7/1, Add Constant6/1, Add Constant5/1, Add Constant4/1, Add Constant3/1, Add Constant13/1, Add Constant14/1
  Gain/1 -> Add/1
  Add Constant/1 -> Gain/1
  Index Vector3/1 -> Add Constant1/1
  Add Constant12/1 -> Mux2/4  "Abril"
  Hora/1 -> Add Constant/1
  Gain2/1 -> y/1
  Gain1/1 -> Gain2/1
  Add/1 -> Gain1/1
  Add Constant4/1 -> Mux2/11  "Noviembre"
  Add Constant3/1 -> Mux2/12  "Diciembre"
  Add Constant5/1 -> Mux2/10  "Octubre"
  Add Constant8/1 -> Mux2/7  "Julio"
  Add Constant13/1 -> Mux2/3  "Marzo"
  Add Constant7/1 -> Mux2/8  "Agosto"
  Mux2/1 -> Index Vector3/2
  Add Constant1/1 -> Add/2
  Add Constant10/1 -> Mux2/5  "Mayo"
  Add Constant14/1 -> Mux2/2  "Febrero"
  Add Constant9/1 -> Mux2/6  "Junio"
  Add Constant6/1 -> Mux2/9  "Septiembre"
  mes/1 -> Index Vector3/1
